simulink model "ex3_s"  (R2018b)
settings: Solver=VariableStepAuto  StartTime=0.0  StopTime=10.0  RelTol=1e-3
values from neighbouring files (symbols this model uses):
  A = [-11 -2.5 0;4 0 0;0 0.25 0]    [ex1.m]    (also in ex2.m; ex3.m = sys_s.a; ex4.m = sys_s.A; ex5.m = sys_c.A)
  B = [4 0 0]'    [ex1.m]    (also in ex2.m; ex3.m = sys_s.b; ex4.m = sys_s.B; ex5.m = sys_c.B)
  C = [0 0 5]    [ex1.m]    (also in ex2.m; ex3.m = sys_s.c; ex4.m = sys_s.C; ex5.m = sys_c.C)
  k_wstar = k_d/k_Fstar    [ex3.m]    (also in ex8.m; motore_posizione.m = k_d/k_F)
  Kstar = -acker(Astar,Bstar,lam_dz)    [ex3.m]    (also in ex8.m; motore_posizione.m = -acker(Astar,Bstar,lam_dstar))
  T = 0.5/20    (= 0.025)    [ex3.m]    (also in ex5.m = 0.1; ex6.m = 0.2; ex8.m = 0.15; motore_posizione.m = 0.3)
settings Model: Creator=hp  LastModifiedBy=michelemaresca
settings DataIOCC: ReturnWorkspaceOutputs=on

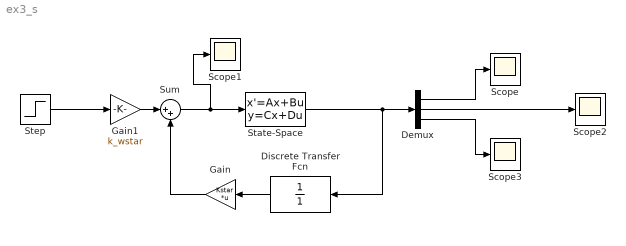
== system ex3_s ==
  Demux : Demux  Outputs=3
  Discrete Transfer Fcn : DiscreteTransferFcn  Denominator=[1]  SampleTime=T
  Gain : Gain  Gain=Kstar  Multiplication=Matrix(K*u)
  Gain1 : Gain  Gain=k_wstar
  Scope{,1..3} (4 alike) : Scope
  State-Space : StateSpace  A=A  B=B  C=[1 0 0;0 1 0;C]  D=zeros(3,1)  InitialCondition=0
  Step : Step  Time=0  SampleTime=T
  Sum : Sum  Inputs=|++
  wires:
  Step/1 -> Gain1/1
  Gain1/1 -> Sum/1
  Sum/1 -> Scope1/1, State-Space/1
  Discrete Transfer Fcn/1 -> Gain/1
  Gain/1 -> Sum/2
  State-Space/1 -> Demux/1, Discrete Transfer Fcn/1
  Demux/1 -> Scope/1
  Demux/3 -> Scope3/1
  Demux/2 -> Scope2/1
